simulink model "MAS_Partial_State_2021a"  (R2021a)
settings: Solver=VariableStepAuto  StartTime=0.0  StopTime=20  RelTol=1e-3
libraries: cstblocks x3
settings Model: Creator=lenovo  LastModifiedBy=lenovo

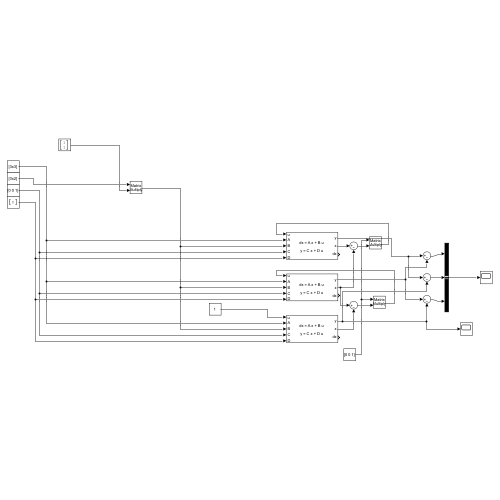
[thumbnail: Simulink's stored preview of the top-level diagram]
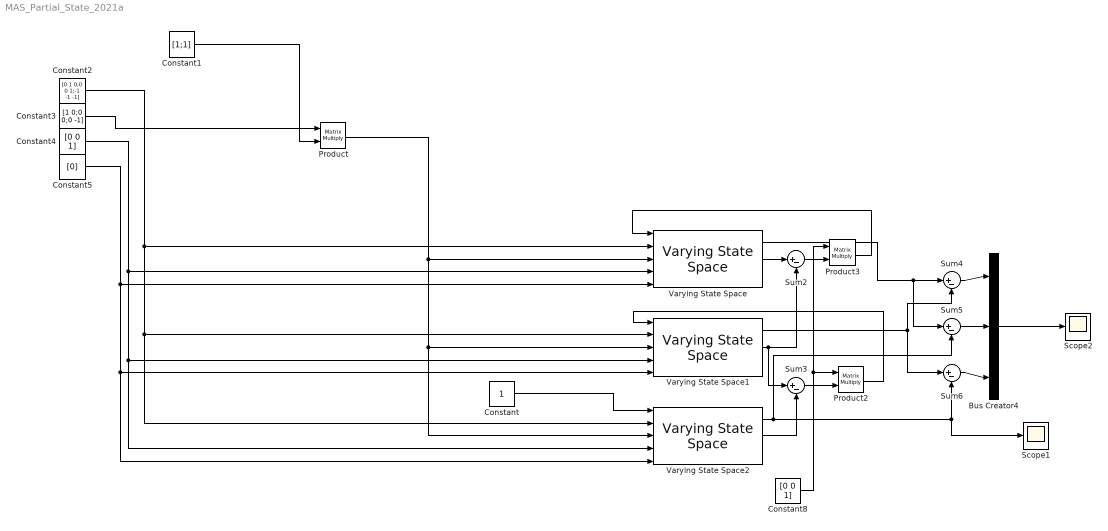
== system MAS_Partial_State_2021a ==
  Bus Creator4 : BusCreator  Inputs=3
  Constant : Constant
  Constant1 : Constant  Value=[1;1]  VectorParams1D=off
  Constant2 : Constant  Value=[0 1 0;0 0 1;-1 -1 -1]
  Constant3 : Constant  Value=[1 0;0 0;0 -1]
  Constant4 : Constant  Value=[0 0 1]  VectorParams1D=off
  Constant5 : Constant  Value=[0]  VectorParams1D=off
  Constant8 : Constant  Value=[0 0 1]  VectorParams1D=off
  Product : Product  Multiplication=Matrix(*)
  Product2 : Product  Multiplication=Matrix(*)
  Product3 : Product  Multiplication=Matrix(*)
  Scope1 : Scope
  Scope2 : Scope
  Sum{2..6} (5 alike) : Sum  Inputs=|+-
  Varying State Space : cstblocks/Linear Parameter Varying/Varying State Space  x0=0  xNames=''  OutputX=on  OutputDX=on
  Varying State Space1 : cstblocks/Linear Parameter Varying/Varying State Space  x0=0  xNames=''  OutputX=on  OutputDX=on
  Varying State Space2 : cstblocks/Linear Parameter Varying/Varying State Space  x0=0  xNames=''  OutputX=on  OutputDX=on
  wires:
  Constant2/1 -> Varying State Space2/2, Varying State Space1/2, Varying State Space/2
  Sum6/1 -> Bus Creator4/3
  Bus Creator4/1 -> Scope2/1
  Sum5/1 -> Bus Creator4/2
  Varying State Space/1 -> Sum5/1, Sum4/1
  Sum4/1 -> Bus Creator4/1
  Varying State Space2/1 -> Sum6/2, Scope1/1, Sum5/2
  Constant3/1 -> Product/1
  Varying State Space/2 -> Sum2/1
  Constant1/1 -> Product/2
  Varying State Space2/2 -> Sum3/2
  Varying State Space1/2 -> Sum2/2, Sum3/1
  Constant5/1 -> Varying State Space2/5, Varying State Space1/5, Varying State Space/5
  Product/1 -> Varying State Space2/3, Varying State Space1/3, Varying State Space/3
  Varying State Space1/1 -> Sum6/1, Sum4/2
  Constant4/1 -> Varying State Space2/4, Varying State Space1/4, Varying State Space/4
  Constant8/1 -> Product2/1, Product3/1
  Sum2/1 -> Product3/2
  Product3/1 -> Varying State Space/1
  Sum3/1 -> Product2/2
  Constant/1 -> Varying State Space2/1
  Product2/1 -> Varying State Space1/1
